simulink model "SemiOffline_DataImport_AND_Preprocessing_ECGandSCG3D"  (R2019a)
settings: Solver=FixedStepDiscrete  StartTime=0.0  StopTime=sim_time + param_frame_size_sec  FixedStep=1/fs  MaxStep=1/fs  RelTol=1e-3
undefined symbols (not defined in the file): fdesignblkfcn, fs, gcbh, param_frame_size_sec, tot_samples
(part 2 of 3)

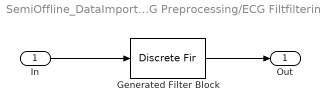
== system SemiOffline_DataImport_AND_Preprocessing_ECGandSCG3D/ECG Preprocessing/ECG Filtfiltering/Bandpass Filter 2 ==
  In : Inport
  Generated Filter Block : DiscreteFir  Tag=BlockMethodSubSystem  Coefficients=[0.000599681428480406667 0.00022427881711320835 0.000262189229493461906 0.000301151231840785058 0.000340510589773355293 0.000379471739139127223 0.000417264520068358531 0.000453028670626539611 0.000485966954942475358 0.00051520760979863558 0.000539947448272285867 0.000559296976009684673 0.000572459856652281327 0.000578602477107202379 0.000577082054079471073 0.000567310721348460796 0.000548962217988804477 0.000521740662199047796 0.000485547849092085506 0.000440237445712871403 0.000385936203776109077 0.0003229072755123711 0.000251933844194426903 0.000173864022162185553 8.96622951676985882e-05 -1.57244866912700784e-07 -9.44856236782579242e-05 -0.000191498736668446122 -0.000288821218832035532 -0.000387533990135975289 -0.000483387582565404498 -0.0005761939607201366 -0.000663970783304963915 -0.000744998643679979622 -0.000817872499416035523 -0.000880964362066854394 -0.000933038029693197195 -0.000972819175774386783 -0.000999391982786898819 -0.00101188643953785775 -0.00100975562147095736 -0.0009925777872959497 -0.000960301557973968888 -0.000913095371979611662 -0.000851475875971816542 -0.000776120817800070653 -0.000687956792167104684 -0.000588107835108653276 -0.000478027414632521848 -0.000359399960207810011 -0.000234020645553201104 -0.000103693767713263781 2.96347327928040449e-05 0.000163739535853423413 0.000296477349825991486 0.000425963905314958593 0.000550271710824708736 0.000666957213482007386 0.000774942628045007312 0.000872177327279355982 0.000957465516398583625 0.00102970621888984269 0.00108791155925947033 0.00113161169633735001 0.00116043044083965412 0.0011744928939702423 0.00117405121060814872 0.00115977134711482406 0.00113246741259064921 0.00109334691797877397 0.00104377213487224217 0.000985398948140998616 0.000919928026674857939 0.000849253670460306097 0.000775309012431770091 0.000700173020871669742 0.000625831434083841767 0.000554224460255208049 0.000487166253492989055 0.000426450533091061459 0.000373619349808891274 0.000329927391772101672 0.000296427775797514052 0.000274047129555466101 0.000263269264543539259 0.000264157227992290519 0.000276874450267364388 0.000300788149948878205 0.000335318317219354277 0.000379524997454130854 0.000432116465419417437 0.000491744413303003814 0.000556678027257966729 0.000625231365131872401 0.000695472120517187306 0.000765547328755601729 0.000833457105991844546 0.000897350978582148358 0.000955377677051596087 0.00100593089701688995 0.00104747392905528316 0.00107875626706505925 0.00109870509459187833 0.00110663185599915856 0.00110205240167736483 0.00108482227065854683 0.00105506279689406663 0.00101332829262456995 0.000960389758015832038 0.000897294817939977879 0.0008253500824062772 0.000746184239515585096 0.000661481098250255592 0.000573117805415166684 0.000483198626351262744 0.000393641448412858244 0.000306548825905859836 0.000223915957856876999 0.000147575494923837179 7.93483670767496796e-05 2.0679134117342313e-05 -2.70568547297773252e-05 -6.2900947686025382e-05 -8.60547436648419054e-05 -9.6171340327614761e-05 -9.31315796396773476e-05 -7.72460981475539256e-05 -4.90464702055338356e-05 -9.48878629550117885e-06 4.02424070543771421e-05 9.86143682268325855e-05 0.000163975772433438543 0.000234396831494164046 0.000307849569477817292 0.000382148726522325442 0.000455178453888958954 0.000524750281940376253 0.000588791425088850046 0.000645337762489050257 0.000692671840552972233 0.000729179983312047068 0.000753614641450886871 0.000765041942292764266 0.000762766365786752784 0.000746540173588745664 0.000716442000586304303 0.000672869753273410646 0.000616693112415834534 0.000548961839282761715 0.000471193538365353938 0.000385043306713752601 0.000292542948292242168 0.000195781895046972886 9.70798634232155033e-05 -1.26466659842236589e-06 -9.68248365214415734e-05 -0.000187315516146842245 -0.000270487917175212054 -0.000344346840215538515 -0.000407012200967724123 -0.000456962738277819839 -0.000492929167971300737 -0.000514057150433395722 -0.000519773775474877196 -0.000509999280888828277 -0.000484990084874355025 ...(+20204 chars)]  InputProcessing=Columns as channels (frame based)
  Out : Outport
  wires:
  Generated Filter Block/1 -> Out/1
  In/1 -> Generated Filter Block/1

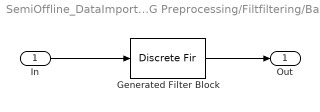
== system SemiOffline_DataImport_AND_Preprocessing_ECGandSCG3D/SCG Preprocessing/Filtfiltering/Bandpass Filter 1 ==
  In : Inport
  Generated Filter Block : DiscreteFir  Tag=BlockMethodSubSystem  Coefficients=[-0.000647770338075434929 -0.000343517502483878777 -0.000420326780186868994 -0.000497874681447326448 -0.000572163883567983742 -0.000640228248060424696 -0.000697341620736447246 -0.000741100378547245487 -0.000767502343489427749 -0.000773945311594367771 -0.000756163673465519263 -0.000715781040457746714 -0.000649518851291922667 -0.000558754413187999722 -0.00044468802672256876 -0.000309569390145499881 -0.000157346999555588955 7.56309344158924597e-06 0.00017981999696271481 0.000352907358331129323 0.000520173062377952814 0.000675059629141158213 0.000810832524492023751 0.000920902297954280416 0.00100022555744028814 0.00104339585916609994 0.00104784075236300563 0.00101082276479851942 0.000932493196038372985 0.00081372483012750324 0.000658118786716569456 0.000469697822827719303 0.000255159625340334827 2.14396010500159063e-05 -0.000222748792724650451 -0.000468614551614006489 -0.000706670354182749056 -0.000927970460822908987 -0.00112339311178654235 -0.00128559051618629583 -0.0014075719529827971 -0.0014847378077428345 -0.00151343561916275301 -0.00149285314374439848 -0.00142321603360264838 -0.00130784430924640264 -0.0011507255600504238 -0.000958682411888284636 -0.000738927946466580573 -0.000500553073942569017 -0.000252448107042536841 -4.51228298674853645e-06 0.000234444470312946134 0.000455461207387870327 0.000651469166657359794 0.000816082599625653801 0.000945275154119637169 0.00103619033374766209 0.00108877327251135801 0.00110401335657345613 0.00108571053871140614 0.00103834647166455344 0.000968694804841021824 0.000883612324176489129 0.00079141959854462133 0.000699633357995322258 0.000616426848716069425 0.000548300984414140311 0.000501481625634690124 0.000479961455332933733 0.000486789456532214109 0.000522442357222020651 0.00058627283270533989 0.000674998416817543592 0.000784500194055535245 0.000908445013836128119 0.00104019836345509912 0.00117163853730648101 0.00129524246150523035 0.00140281134401658617 0.00148771616471947161 0.00154348036758589994 0.00156593860019076754 0.00155180420574065276 0.00150047956618671327 0.0014125221351874741 0.00129124537708533681 0.00114095226621692479 0.000968283947858580374 0.000780347697060279968 0.00058580174682495306 0.000392949669008726315 0.000210739838125063969 4.67353233640661067e-05 -9.17098537984661032e-05 -0.000199474799964817527 -0.000272369167151098905 -0.000308956715154304199 -0.000309062680725871372 -0.000275382856037888104 -0.000211718414908937836 -0.00012440394301087011 -2.03462178716174195e-05 9.18365595282383371e-05 0.000203774330319042617 0.000306382694897032286 0.00039183217102360077 0.000452554892511169168 0.000483155558882161773 0.000479279720088677912 0.000439316668050006678 0.000363105403623313172 0.000253394761208263191 0.000114230004232997954 -4.77446668554886442e-05 -0.000225181088213468402 -0.000408917488377553637 -0.000589991911142579025 -0.00075869987196111393 -0.000906593394805637102 -0.00102553663011526602 -0.00110963698146597858 -0.00115418825375746253 -0.00115734164105921774 -0.00111890913599901019 -0.00104171557147943856 -0.000930164097664520385 -0.000791336524032147009 -0.000633259801675410032 -0.000465832430360793397 -0.000298919925422787205 -0.000143130722921475659 -7.86877071387343148e-06 9.78644949485511892e-05 0.000167363222362294718 0.00019525861251619436 0.000179203991855867199 0.000118725167489869548 1.6541729219412952e-05 -0.000122793742983712804 -0.000291899772648228362 -0.000482194263276236991 -0.000683150339584172187 -0.00088409319788581046 -0.00107362450916950779 -0.00124144751215223763 -0.00137781033119710916 -0.00147526394058089061 -0.00152791278658659293 -0.00153299420877785588 -0.00148987526532067937 -0.00140130121930216343 -0.00127211455353073055 -0.00111015084855621581 -0.000924679192769932478 -0.000727023678111190933 -0.000528801782353420513 -0.000342348805686419622 -0.00017894991212643208 -4.92046497649435222e-05 3.86290643596606527e-05 7.81216788691107265e-05 6.61062040557425386e-05 1.87789399799218092e-06 -0.000111703526733958531 ...(+15232 chars)]  InputProcessing=Columns as channels (frame based)
  Out : Outport
  wires:
  Generated Filter Block/1 -> Out/1
  In/1 -> Generated Filter Block/1
